simulink model "CAVE_MachE_dSPACE_250912"  (R2024a)
settings: configuration reference "ConfigSetDesktopFixedStep" (kept outside this file)
PreLoadFcn:
  | VSS_BICYCLE=Simulink.Variant('Dual=0');
  | VSS_DUAL=Simulink.Variant('Dual=1');
  | Dual=1;
  | load('DriveCycle2.mat')
PostLoadFcn:
  | if any(exist('dsrtsu_mdlpostloadfcn', 'file') ~= 0), dsrtsu_mdlpostloadfcn('Execute', bdroot); end
InitFcn:
  | , if any(exist('rtifpga_mdlclblib', 'file') ~= 0), rtifpga_mdlclblib('Init', bdroot); end,
  | , if any(exist('dsmpb_private', 'file') ~= 0), dsmpb_private('dsmpb_mdlclblib', 'Init', bdroot); end,
  | load('DriveCycle2.mat')
model workspace (MAT data in the model file):
  Gas = 0.383333333333
values from neighbouring files (symbols this model uses):
  CoastDown =     [Run_Simulink.mat]
  limitedMCT =     [Run_Simulink.mat]
  MCT =     [Run_Simulink.mat]
  pMCT =     [Run_Simulink.mat]
  RealSimPara =     [Run_Simulink.mat]
  Ref_speed = [13 13.007895099 13.015778396 13.023649891 13.031509584 13.039357475 13.047193564 13.055017851 13.062830336 13.070631019 13.0784199 13.086196979 ... (2669 elements, 2669x1)]    [Ref_speed_and_time.mat]
  Ref_time = [0 0.01 0.02 0.03 0.04 0.05 0.06 0.07 0.08 0.09 0.1 0.11 ... (2669 elements, 2669x1)]    [Ref_speed_and_time.mat]
  US06 =     [Run_Simulink.mat]
undefined symbols (not defined in the file or in its folder): AccelCmd, ActTqLF_Nm_, ActTqLR_Nm_, ActTqRF_Nm_, ActTqRR_Nm_, BattChargeLimitMaxPwr, BattChargeLimitSocBpts, BattChargeLimitTbl, BattChrgCapcty, BattDischargeLimitSocBpts, BattDischargeLimitTbl, BattDischargeMaxPwr, BattNumCellsParallel, BattNumCellsSeries, BattOpenVoltCapBpts, BattOpenVoltTbl, BattResistSocBpts, BattResistTbl, BattResistTempBpts, BrakeMaxPrs, BrakeMaxTrq, ChassisDistCg2FrontAxle, ChassisDistCg2RearAxle, ChassisVehMass, CltchCmd, DecelCmd, DiffRatio, DiscIntNeverNeededParam, EnvGravCnst, EnvPrs, EnvTemp, FuelSpecificGrav, GearCmd, h, InitStates, lgSw, MtrEffSpdBpts, MtrEffTbl, MtrEffTrqBpts, MtrPwrMax, MtrTrqMax, SteeringCmd, SupvsryCtrlRegenBrkCutOffTbl, SupvsryCtrlRegenSpdBpts, TestScnrioCycleNum, VEH
libraries: VSIGenLib x122, simulink x112, etargetslib x75, dsmpblib x55, vehdynlibtire x24, CarMaker4SL x20, autolibshared x19, vehdynlibsuspension x14, vehdynlibtirecommon x14, autolibutils x10, VsrLibWheel x8, autolibpowerinfoutils x6
(part 15 of 31)

== system CAVE_MachE_dSPACE_250912/Vehicle Under Test2/Vehicle/Vehicle Dynamics/Vehicle 7DOF/Longitudinal Wheels 4DOF/Tires ==
  AxlTrq : Inport
  BrkPrs : Inport  Port=2
  Vx : Inport  Port=3
  Vy : Inport  Port=4
  r : Inport  Port=5
  Camber : Inport  Port=6
  TirePrs : Inport  Port=7
  Fz : Inport  Port=8
  lam_mu : Inport  Port=9
  Gnd : Inport  Port=10
  4-by-1 Gnd : Subsystem
  4-by-1 Gnd1 : Subsystem
  4-by-1 Gnd2 : Subsystem
  4-by-1 Gnd3 : Subsystem
  Bus Creator : BusCreator  Inputs=12
  Subsystem : Subsystem
  Terminator1 : Terminator
  Terminator2 : Terminator
  Terminator3 : Terminator
  Wheel : Outport  VectorParamsAs1DForOutWhenUnconnected=off
  wires:
  Vy/1 -> Terminator1/1
  Camber/1 -> Terminator2/1
  r/1 -> Terminator3/1
  Bus Creator/1 -> Wheel/1
  Subsystem/7(zdot) -> Bus Creator/10  "zdot"
  Subsystem/6(z) -> Bus Creator/9  "z"
  Subsystem/2(Fx) -> Bus Creator/2  "Fx"
  Subsystem/1(Omega) -> Bus Creator/1  "Omega"
  Subsystem/5(Re) -> Bus Creator/8  "Re"
  Subsystem/3(FzOut) -> Bus Creator/4  "Fz"
  Subsystem/4(My) -> Bus Creator/6  "My"
  4-by-1 Gnd/1(Gnd) -> Bus Creator/3  "Fy"
  4-by-1 Gnd1/1(Gnd) -> Bus Creator/5  "Mx"
  4-by-1 Gnd2/1(Gnd) -> Bus Creator/7  "Mz"
  Subsystem/8(Kappa) -> Bus Creator/11  "Kappa"
  4-by-1 Gnd3/1(Gnd) -> Bus Creator/12  "Alpha"
  AxlTrq/1 -> Subsystem/1(AxlTrq)
  BrkPrs/1 -> Subsystem/2(BrkPrs)
  Vx/1 -> Subsystem/3(Vx)
  TirePrs/1 -> Subsystem/4(TirePrs)
  Fz/1 -> Subsystem/5(Fz)
  lam_mu/1 -> Subsystem/6(lam_mu)
  Gnd/1 -> Subsystem/7(Gnd)

== system CAVE_MachE_dSPACE_250912/Vehicle Under Test2/Vehicle/Vehicle Dynamics/Vehicle 7DOF/Longitudinal Wheels 4DOF/Veh2Tire ==
  AxlTrq : Inport
  BrkPrs : Inport  Port=2
  r : Inport  Port=3
  VehVel : Inport  Port=4
  WhlAng : Inport  Port=5
  Reshape3 : Reshape
  Reshape4 : Reshape
  Unary Minus : UnaryMinus
  Wheel to Body Transform : Subsystem
  T : Outport  VectorParamsAs1DForOutWhenUnconnected=off
  P : Outport  Port=2  VectorParamsAs1DForOutWhenUnconnected=off
  xdotAxle : Outport  Port=3  VectorParamsAs1DForOutWhenUnconnected=off
  ydotAxle : Outport  Port=4  VectorParamsAs1DForOutWhenUnconnected=off
  psidot : Outport  Port=5  VectorParamsAs1DForOutWhenUnconnected=off
  zdotAxle : Outport  Port=6  VectorParamsAs1DForOutWhenUnconnected=off
  wires:
  BrkPrs/1 -> Reshape3/1
  AxlTrq/1 -> Reshape4/1
  Wheel to Body Transform/1(xdotWheel) -> xdotAxle/1  "Vx"
  Wheel to Body Transform/2(ydotWheel) -> ydotAxle/1  "Vy"
  r/1 -> Unary Minus/1
  Reshape4/1 -> T/1
  VehVel/1 -> Wheel to Body Transform/1(VelVeh)
  WhlAng/1 -> Wheel to Body Transform/2(WhlAng)
  Wheel to Body Transform/3(zdotWheel) -> zdotAxle/1  "Vz"
  Unary Minus/1 -> psidot/1
  Reshape3/1 -> P/1

== system CAVE_MachE_dSPACE_250912/Vehicle Under Test2/Vehicle/Vehicle Dynamics/Vehicle 7DOF/Longitudinal Wheels 4DOF/Velocity and Vertical Load ==
  note: 1) Add Subsystem or Model blocks as valid variant choices.
      | 2) You cannot connect blocks at this level. At simulation, connectivity is automatically
      | determined, based on the active variant and port name matching.
  VehFdbk : Inport
  Bicycle : Subsystem  VariantControl=0
  Dual : Subsystem  VariantControl=1
  VehVel : Outport  VectorParamsAs1DForOutWhenUnconnected=off
  Fz : Outport  Port=2  PortDimensions=4  VectorParamsAs1DForOutWhenUnconnected=off

== system CAVE_MachE_dSPACE_250912/Vehicle Under Test2/Vehicle/Vehicle Dynamics/Vehicle 7DOF/Longitudinal Wheels 4DOF/Wheel Angles ==
  WheelAng : Inport
  Camber : Inport  Port=2
  Add1 : Sum
  Constant2 : Constant  Value=0
  Constant3 : Constant  Value=ones(1,4).*pi
  Demux : Demux  Outputs=2
  Demux1 : Demux
  Mux : Mux  Inputs=2
  Reshape : Reshape  OutputDimensionality=Row vector (2-D)
  Reshape1 : Reshape  OutputDimensionality=Row vector (2-D)
  Reshape2 : Reshape  OutputDimensionality=Row vector (2-D)
  Vector Concatenate3 : Concatenate  NumInputs=3  Mode=Multidimensional array
  Vector Concatenate4 : Concatenate  NumInputs=4
  WhlAngB : Outport  VectorParamsAs1DForOutWhenUnconnected=off
  wires:
  Demux1/2 -> Mux/1
  Constant2/1 -> Add1/2
  Add1/1 -> Demux/1
  Demux1/3 -> Vector Concatenate4/3
  Demux1/1 -> Vector Concatenate4/1
  Mux/1 -> Add1/1
  Demux1/4 -> Mux/2
  Demux/1 -> Vector Concatenate4/2
  Demux/2 -> Vector Concatenate4/4
  Vector Concatenate4/1 -> Reshape/1
  Constant3/1 -> Reshape1/1
  Vector Concatenate3/1 -> WhlAngB/1
  Reshape/1 -> Vector Concatenate3/3
  Reshape1/1 -> Vector Concatenate3/1
  Reshape2/1 -> Vector Concatenate3/2
  Camber/1 -> Reshape2/1
  WheelAng/1 -> Demux1/1

== system CAVE_MachE_dSPACE_250912/Vehicle Under Test2/Vehicle/Vehicle Dynamics/Vehicle 7DOF/Subsystem4/Subsystem ==
  CgXYZdot : Inport
  angles : Inport  Port=2
  Demux2 : Demux  Outputs=3
  Demux3 : Demux  Outputs=3
  Terminator{,1..4} (5 alike) : Terminator
  VehSpd : Outport
  wires:
  CgXYZdot/1 -> Demux2/1
  Demux3/2 -> Terminator3/1  "theta"
  Demux2/2 -> Terminator/1  "Ydot"
  Demux3/1 -> Terminator2/1  "phi"
  Demux3/3 -> Terminator4/1  "psi"
  Demux2/3 -> Terminator1/1  "Zdot"
  angles/1 -> Demux3/1
  Demux2/1 -> VehSpd/1  "Xdot"

== system CAVE_MachE_dSPACE_250912/Vehicle Under Test2/Vehicle/Vehicle Dynamics/Vehicle 7DOF/Vehicle Body 3DOF External Longitudinal Wheels/Bicycle ==
  WhlAng : Inport
  "FwF " : Inport  Port=2
  "FwR " : Inport  Port=3
  WindXYZ : Inport  Port=4
  Friction : Inport  Port=5
  Demux : Demux  Outputs=[2,2]
  Gain : Gain  Gain=.5
  Gain1 : Gain  Gain=.5
  Gain2 : Gain  Gain=.5
  Selector : Selector  InputPortWidth=4  IndexOptions=Index vector (dialog)  Indices=[1 2]  OutputSizes=1
  Signal Specification : SignalSpecification  Unit=1
  Signal Specification1 : SignalSpecification  Unit=rad
  Sum of Elements : Sum  Inputs=+
  Sum of Elements1 : Sum  Inputs=+
  Sum of Elements2 : Sum  Inputs=+
  Terminator{,1..5} (6 alike) : Terminator
  Vector Concatenate : Concatenate
  Vehicle Body 3DOF Single Track : autolibshared/Vehicle Body 3DOF Single Track  trackMode=Single (bicycle)  inputMode=External longitudinal forces  frontSteerMode=on  rearSteerMode=off  windMode=on  muMode=on  extFMode=off  extMMode=off  htchFMode=off  htchMMode=off  extXo=off  extpsio=off  extxdoto=off  extro=off  extYo=off  extTamb=off  extydoto=off  aMode=2  NF=ChassisNumFrontWhls  NR=ChassisNumRearWhls  m=ChassisVehMass  a=ChassisDistCg2FrontAxle  b=ChassisDistCg2RearAxle  h=ChassisCgHeight  dh=1  hh=0.2  X_o=0  xdot_o=20  CalphaMode=off  sigmaMode=on  d=0  hl=0  w=1.922.*[1 1]  Cy_f=15000  Cy_r=35000  sigma_f=.1  sigma_r=.1  alpha_f_brk=[-.1 .1]  Cy_f_data=[-9e3 9e3]  alpha_r_brk=[-.1 .1]  Cy_r_data=[-9e3 9e3]  Y_o=0  ydot_o=0  Izz=2500  psi_o=0  r_o=0  Af=ChassisFrontalArea  Cd=ChassisDragCoeff  Cl=.1  Cpm=.1  beta_w=[0:0.01:0.3]  Cs=[0:0.03:0.9]  Cym=[0:0.01:0.3]  Pabs=EnvPrs  Tair=EnvTemp  g=EnvGravCnst  mu=1  xdot_tol=1  Fznom=5000  Fxtire_sat=7e3*1e3  Fytire_sat=2e3*1e3  longOff=0  latOff=0  vertOff=.0112  wrapAng=off
  Wheel Positions : Subsystem
  " Info" : Outport  VectorParamsAs1DForOutWhenUnconnected=off
  XWheel : Outport  Port=2  Unit=m  VectorParamsAs1DForOutWhenUnconnected=off
  " YWheel" : Outport  Port=3  Unit=m  VectorParamsAs1DForOutWhenUnconnected=off
  wires:
  "FwR "/1 -> Vehicle Body 3DOF Single Track/3
  "FwF "/1 -> Vehicle Body 3DOF Single Track/2
  Vehicle Body 3DOF Single Track/1 -> " Info"/1, Wheel Positions/1(Info)
  WhlAng/1 -> Selector/1
  Gain/1 -> Signal Specification1/1
  Sum of Elements/1 -> Gain/1
  Vehicle Body 3DOF Single Track/6 -> Terminator/1
  Vehicle Body 3DOF Single Track/7 -> Terminator1/1
  WindXYZ/1 -> ?
  Selector/1 -> Sum of Elements/1
  Demux/1 -> Sum of Elements1/1
  Friction/1 -> Demux/1
  Sum of Elements1/1 -> Gain1/1
  Sum of Elements2/1 -> Gain2/1
  Demux/2 -> Sum of Elements2/1
  Gain1/1 -> Vector Concatenate/1
  Gain2/1 -> Vector Concatenate/2
  Vector Concatenate/1 -> Signal Specification/1
  Signal Specification/1 -> ?
  Signal Specification1/1 -> Vehicle Body 3DOF Single Track/1
  Wheel Positions/2(YWheel) -> " YWheel"/1
  Wheel Positions/1(XWheel) -> XWheel/1
  Vehicle Body 3DOF Single Track/4 -> Terminator2/1
  Vehicle Body 3DOF Single Track/5 -> Terminator3/1
  Vehicle Body 3DOF Single Track/2 -> Terminator4/1
  Vehicle Body 3DOF Single Track/3 -> Terminator5/1

== system CAVE_MachE_dSPACE_250912/Vehicle Under Test2/Vehicle/Vehicle Dynamics/Vehicle 7DOF/Vehicle Body 3DOF External Longitudinal Wheels/Dual ==
  WhlAng : Inport
  "FwF " : Inport  Port=2
  "FwR " : Inport  Port=3
  WindXYZ : Inport  Port=4
  Friction : Inport  Port=5
  Reshape : Reshape  OutputDimensionality=Customize  OutputDimensions=[2,2]
  Selector : Selector  InputPortWidth=4  IndexOptions=Index vector (dialog)  Indices=[1 2]  OutputSizes=1
  Signal Specification : SignalSpecification  Unit=1
  Terminator{,1..5} (6 alike) : Terminator
  Vehicle Body 3DOF Dual Track : autolibshared/Vehicle Body 3DOF Single Track  trackMode=Dual  inputMode=External longitudinal forces  frontSteerMode=on  rearSteerMode=off  windMode=on  muMode=on  extFMode=off  extMMode=off  htchFMode=off  htchMMode=off  extXo=off  extpsio=off  extxdoto=off  extro=off  extYo=off  extTamb=off  extydoto=off  aMode=2  NF=ChassisNumFrontWhls  NR=ChassisNumRearWhls  m=ChassisVehMass  a=ChassisDistCg2FrontAxle  b=ChassisDistCg2RearAxle  h=ChassisCgHeight  dh=1  hh=0.2  X_o=0  xdot_o=InitStates(TestScnrioCycleNum).VehSpd  CalphaMode=off  sigmaMode=on  d=0  hl=0  w=1.9.*[1 1]  Cy_f=15000  Cy_r=35000  sigma_f=.1  sigma_r=.1  alpha_f_brk=[-.1 .1]  Cy_f_data=[-9e3 9e3]  alpha_r_brk=[-.1 .1]  Cy_r_data=[-9e3 9e3]  Y_o=0  ydot_o=0  Izz=2500  psi_o=0  r_o=0  Af=ChassisFrontalArea  Cd=ChassisDragCoeff  Cl=.1  Cpm=.1  beta_w=[0:0.01:0.3]  Cs=[0:0.03:0.9]  Cym=[0:0.01:0.3]  Pabs=EnvPrs  Tair=EnvTemp  g=EnvGravCnst  mu=1  xdot_tol=1  Fznom=5000  Fxtire_sat=7e3*1e3  Fytire_sat=2e3*1e3  longOff=0  latOff=0  vertOff=.0112  wrapAng=off
  Wheel Positions : Subsystem
  " Info" : Outport  VectorParamsAs1DForOutWhenUnconnected=off
  " XWheel" : Outport  Port=2  VectorParamsAs1DForOutWhenUnconnected=off
  " YWheel" : Outport  Port=3  VectorParamsAs1DForOutWhenUnconnected=off
  wires:
  WhlAng/1 -> Selector/1
  Selector/1 -> Vehicle Body 3DOF Dual Track/1
  Friction/1 -> Reshape/1
  Reshape/1 -> Signal Specification/1
  Vehicle Body 3DOF Dual Track/1 -> " Info"/1, Wheel Positions/1(Info)
  Wheel Positions/1(XWheel) -> " XWheel"/1
  Wheel Positions/2(YWheel) -> " YWheel"/1
  Vehicle Body 3DOF Dual Track/2 -> Terminator4/1
  Vehicle Body 3DOF Dual Track/3 -> Terminator5/1
  Vehicle Body 3DOF Dual Track/6 -> Terminator1/1
  Vehicle Body 3DOF Dual Track/4 -> Terminator2/1
  Vehicle Body 3DOF Dual Track/5 -> Terminator3/1
  Vehicle Body 3DOF Dual Track/7 -> Terminator/1
  Signal Specification/1 -> ?
  WindXYZ/1 -> ?
  "FwF "/1 -> Vehicle Body 3DOF Dual Track/2
  "FwR "/1 -> Vehicle Body 3DOF Dual Track/3

== system CAVE_MachE_dSPACE_250912/Vehicle Under Test2/Vehicle/Vehicle Dynamics/Vehicle Longitudinal/Longitudinal Wheels/Front Diff Wheels ==
  BrkPrs : Inport
  AxleTorq : Inport  Port=2
  Add2 : Sum
  Bus Creator : BusCreator  Inputs=3
  Bus Creator5 : BusCreator  Inputs=1
  Bus Selector6 : BusSelector  OutputSignals=VehSpd,FrcZ
  Bus Selector7 : BusSelector  OutputSignals=VehSpd,FrcZ
  Selector : Selector  InputPortWidth=4  IndexOptions=Index vector (dialog)  Indices=1  OutputSizes=1
  Selector1 : Selector  InputPortWidth=4  IndexOptions=Index vector (dialog)  Indices=2  OutputSizes=1
  Selector2 : Selector  InputPortWidth=4  IndexOptions=Index vector (dialog)  Indices=1  OutputSizes=1
  Selector3 : Selector  InputPortWidth=4  IndexOptions=Index vector (dialog)  Indices=2  OutputSizes=1
  Simple Longitudinal Wheel 1 : VsrLibWheel/Simple Longitudinal Wheel  TireLoadedRadius=WhlRearLoadedRadius  C_rr=WhlRollingResistCnst  MaxBrkTrq=BrakeMaxTrq  MaxBrkPrs=BrakeMaxPrs  w_thresh=WhlSimVelTol
  Simple Longitudinal Wheel 2 : VsrLibWheel/Simple Longitudinal Wheel  TireLoadedRadius=WhlRearLoadedRadius  C_rr=WhlRollingResistCnst  MaxBrkTrq=BrakeMaxTrq  MaxBrkPrs=BrakeMaxPrs  w_thresh=WhlSimVelTol
  Terminator3 : Terminator
  Two-Way Connection6 : TwoWayConnection
  DiffAxle : PMIOPort  Side=Right
  Info : Outport
  wires:
  Bus Selector6/2 -> Simple Longitudinal Wheel 1/4  "<FrcZ>"
  BrkPrs/1 -> Selector3/1, Selector2/1
  Simple Longitudinal Wheel 1/2 -> Add2/1
  Bus Selector7/1 -> Simple Longitudinal Wheel 2/3  "<VehSpd>"
  Bus Selector6/1 -> Simple Longitudinal Wheel 1/3  "<VehSpd>"
  Bus Selector7/2 -> Simple Longitudinal Wheel 2/4  "<FrcZ>"
  Two-Way Connection6/1 -> Bus Selector7/1, Bus Selector6/1
  Add2/1 -> Bus Creator5/1  "FrcX"
  Simple Longitudinal Wheel 2/2 -> Add2/2  "Spd"
  Bus Creator5/1 -> Two-Way Connection6/1
  Simple Longitudinal Wheel 2/1 -> Terminator3/1
  Selector2/1 -> Simple Longitudinal Wheel 1/1
  AxleTorq/1 -> Selector1/1, Selector/1
  Selector/1 -> Simple Longitudinal Wheel 1/2
  Selector1/1 -> Simple Longitudinal Wheel 2/2
  Selector3/1 -> Simple Longitudinal Wheel 2/1
  Simple Longitudinal Wheel 1/3 -> Bus Creator/2  "Omega1"
  Bus Creator/1 -> Info/1
  Simple Longitudinal Wheel 1/1 -> Bus Creator/1  "WhlFrontInfo"
  Simple Longitudinal Wheel 2/3 -> Bus Creator/3  "Omega2"
  connections:
  DiffAxle/RConn1 -- Two-Way Connection6/RConn1

== system CAVE_MachE_dSPACE_250912/Vehicle Under Test2/Vehicle/Vehicle Dynamics/Vehicle Longitudinal/Longitudinal Wheels/Rear Wheels ==
  BrkPrs : Inport
  Add2 : Sum
  Bus Creator : BusCreator  Inputs=3
  Bus Creator5 : BusCreator  Inputs=1
  Bus Selector6 : BusSelector  OutputSignals=VehSpd,FrcZ
  Bus Selector7 : BusSelector  OutputSignals=VehSpd,FrcZ
  Ground : Ground
  Selector : Selector  InputPortWidth=4  IndexOptions=Index vector (dialog)  Indices=3  OutputSizes=1
  Selector1 : Selector  InputPortWidth=4  IndexOptions=Index vector (dialog)  Indices=4  OutputSizes=1
  Simple Longitudinal Wheel : VsrLibWheel/Simple Longitudinal Wheel  TireLoadedRadius=WhlFrontLoadedRadius  C_rr=WhlRollingResistCnst  MaxBrkTrq=BrakeMaxTrq  MaxBrkPrs=BrakeMaxPrs  w_thresh=WhlSimVelTol
  Simple Longitudinal Wheel1 : VsrLibWheel/Simple Longitudinal Wheel  TireLoadedRadius=WhlFrontLoadedRadius  C_rr=WhlRollingResistCnst  MaxBrkTrq=BrakeMaxTrq  MaxBrkPrs=BrakeMaxPrs  w_thresh=WhlSimVelTol
  Terminator3 : Terminator
  Two-Way Connection6 : TwoWayConnection
  DiffAxle : PMIOPort  Side=Right
  Info : Outport
  wires:
  Simple Longitudinal Wheel1/1 -> Terminator3/1
  Simple Longitudinal Wheel1/3 -> Bus Creator/3  "Omega4"
  Ground/1 -> Simple Longitudinal Wheel/2, Simple Longitudinal Wheel1/2
  Simple Longitudinal Wheel/3 -> Bus Creator/2  "Omega3"
  Bus Creator5/1 -> Two-Way Connection6/1
  Simple Longitudinal Wheel1/2 -> Add2/2  "Spd"
  Add2/1 -> Bus Creator5/1  "FrcX"
  Two-Way Connection6/1 -> Bus Selector7/1, Bus Selector6/1
  Bus Selector7/2 -> Simple Longitudinal Wheel1/4  "<FrcZ>"
  Bus Selector6/1 -> Simple Longitudinal Wheel/3  "<VehSpd>"
  Bus Selector7/1 -> Simple Longitudinal Wheel1/3  "<VehSpd>"
  Simple Longitudinal Wheel/2 -> Add2/1
  BrkPrs/1 -> Selector1/1, Selector/1
  Bus Selector6/2 -> Simple Longitudinal Wheel/4  "<FrcZ>"
  Selector/1 -> Simple Longitudinal Wheel/1
  Selector1/1 -> Simple Longitudinal Wheel1/1
  Simple Longitudinal Wheel/1 -> Bus Creator/1  "WhlRearInfo"
  Bus Creator/1 -> Info/1
  connections:
  DiffAxle/RConn1 -- Two-Way Connection6/RConn1

== system CAVE_MachE_dSPACE_250912/Vehicle Under Test2/Vehicle/Vehicle Dynamics/Vehicle Longitudinal/Vehicle Body/Logitudinal Vehicle Body ==
  RoadGrade : Inport
  WindVel : Inport  Port=2  Unit=m/s
  Bus Creator : BusCreator  Inputs=2
  Bus Creator1 : BusCreator  Inputs=2
  Bus Selector : BusSelector  OutputSignals=FrcX
  Bus Selector1 : BusSelector  OutputSignals=BdyFrm.Cg.Vel.xdot,BdyFrm.Cg.Disp.x
  Bus Selector3 : BusSelector  OutputSignals=FrcX
  Signal Specification3 : SignalSpecification  Unit=N
  Signal Specification4 : SignalSpecification  Unit=N
  Transfer Fcn : TransferFcn  Denominator=[0.01 1]
  Transfer Fcn1 : TransferFcn  Denominator=[0.01 1]
  Two-Way Connection2 : TwoWayConnection
  Two-Way Connection8 : TwoWayConnection
  Unit Conversion : UnitConversion
  Vehicle Body 1DOF Longitudinal : autolibshared/Vehicle Body 1DOF Longitudinal  VariantControl=SL  extFMode=off  extMMode=off  extTamb=off  wind3D=off  aMode=1  NF=ChassisNumFrontWhls  NR=ChassisNumRearWhls  m=ChassisVehMass  a=ChassisDistCg2FrontAxle  b=ChassisDistCg2RearAxle  h=ChassisCgHeight  Cd=ChassisDragCoeff  Cl=0  Cpm=0  Af=ChassisFrontalArea  x_o=0  xdot_o=InitStates(TestScnrioCycleNum).VehSpd  Pabs=EnvPrs  T=EnvTemp  g=EnvGravCnst
      settings: LibrarySourceBlock=autolibvehdynlong/Vehicle Body 1DOF Longitudinal
  Front : PMIOPort  Side=Left
  Rear : PMIOPort  Port=2  Side=Left
  VehSpd : Outport  VectorParamsAs1DForOutWhenUnconnected=off
  VehDist : Outport  Port=2  VectorParamsAs1DForOutWhenUnconnected=off
  FrontAxleFrc : Outport  Port=3  VectorParamsAs1DForOutWhenUnconnected=off
  RearAxleFrc : Outport  Port=4  VectorParamsAs1DForOutWhenUnconnected=off
  wires:
  Two-Way Connection8/1 -> Bus Selector/1
  RoadGrade/1 -> Unit Conversion/1
  Bus Selector/1 -> Transfer Fcn1/1  "<FrcX>"
  Vehicle Body 1DOF Longitudinal/2 -> Bus Creator/1, Bus Creator1/1  "VehSpd"
  Vehicle Body 1DOF Longitudinal/1 -> Bus Selector1/1  "Veh"
  Signal Specification3/1 -> RearAxleFrc/1, Vehicle Body 1DOF Longitudinal/2  "RearAxleFrc"
  Bus Creator/1 -> Two-Way Connection8/1
  Vehicle Body 1DOF Longitudinal/3 -> Bus Creator/2  "FrcZ"
  WindVel/1 -> Vehicle Body 1DOF Longitudinal/4
  Two-Way Connection2/1 -> Bus Selector3/1
  Vehicle Body 1DOF Longitudinal/4 -> Bus Creator1/2  "FrcZ"
  Bus Selector1/1 -> VehSpd/1  "<xdot>"
  Bus Selector1/2 -> VehDist/1  "<x>"
  Unit Conversion/1 -> Vehicle Body 1DOF Longitudinal/3
  Signal Specification4/1 -> FrontAxleFrc/1, Vehicle Body 1DOF Longitudinal/1  "FrontAxleFrc"
  Transfer Fcn/1 -> Signal Specification3/1
  Transfer Fcn1/1 -> Signal Specification4/1
  Bus Creator1/1 -> Two-Way Connection2/1
  Bus Selector3/1 -> Transfer Fcn/1  "<FrcX>"
  connections:
  Two-Way Connection8/RConn1 -- Front/RConn1
  Two-Way Connection2/RConn1 -- Rear/RConn1

== system CAVE_MachE_dSPACE_250912/Vehicle Under Test2/Vehicle/Vehicle Dynamics/Vehicle Longitudinal/Vehicle Body/Subsystem1 ==
  VehSpd : Inport
  VehDist : Inport  Port=2
  FrontAxleFrc : Inport  Port=3
  RearAxleFrc : Inport  Port=4
  Bus Creator : BusCreator  Inputs=4
  ChassisPlant : Outport
  wires:
  VehSpd/1 -> Bus Creator/1  "VehSpd"
  VehDist/1 -> Bus Creator/2  "VehDist"
  Bus Creator/1 -> ChassisPlant/1  "ChassisPlant"
  FrontAxleFrc/1 -> Bus Creator/3  "FrontAxleFrc"
  RearAxleFrc/1 -> Bus Creator/4  "RearAxleFrc"

== system CAVE_MachE_dSPACE_250912/Vehicle Under Test3/Vehicle/Actuation and Outputs/MOOG Brake Actuator/ CAN Settings/ CAN diagnostic Counter ==
  RX Counter : Inport
  Compare To Constant3 : simulink/Logic and Bit Operations/Compare To Constant  relop=<=  const=TimeOutDuration  OutDataTypeStr=boolean
  Memory2 : Memory  InheritSampleTime=on
  Relational Operator2 : RelationalOperator  Operator=~=  OutDataTypeStr=boolean  InputSameDT=off
  Timer : Subsystem
  CommsOKFlag : Outport
  wires:
  Relational Operator2/1 -> Timer/1(Reset)
  Timer/1(Timer) -> Compare To Constant3/1
  RX Counter/1 -> Relational Operator2/1, Memory2/1
  Memory2/1 -> Relational Operator2/2
  Compare To Constant3/1 -> CommsOKFlag/1

== system CAVE_MachE_dSPACE_250912/Vehicle Under Test3/Vehicle/Actuation and Outputs/MOOG Brake Actuator/MOOG Interface/Max Stop Adjustment ==
  In1 : Inport
  Enable : EnablePort
  MaxStopOffset : Constant  Value=-5500
  Sum3 : Sum  Inputs=|++
  Out1 : Outport  InitialOutput=[0]
  wires:
  MaxStopOffset/1 -> Sum3/2
  In1/1 -> Sum3/1
  Sum3/1 -> Out1/1

== system CAVE_MachE_dSPACE_250912/Vehicle Under Test3/Vehicle/Actuation and Outputs/MOOG Brake Actuator/MOOG Interface/Min Stop Adjustment ==
  In1 : Inport
  Enable : EnablePort
  MinStopOffset : Constant  Value=3500
  Sum3 : Sum  Inputs=|++
  Out1 : Outport  InitialOutput=[0]
  wires:
  In1/1 -> Sum3/1
  Sum3/1 -> Out1/1
  MinStopOffset/1 -> Sum3/2

== system CAVE_MachE_dSPACE_250912/Vehicle Under Test3/Vehicle/Actuation and Outputs/MOOG Brake Actuator/MOOG Interface/Rising edge ==
  In : Inport
  Memory : Memory  InheritSampleTime=on
  Sum3 : Sum  Inputs=|+-
  Out : Outport
  wires:
  In/1 -> Memory/1, Sum3/1
  Memory/1 -> Sum3/2
  Sum3/1 -> Out/1

== system CAVE_MachE_dSPACE_250912/Vehicle Under Test3/Vehicle/Actuation and Outputs/MOOG Brake Actuator/MOOG Interface/Rising edge1 ==
  In : Inport
  Memory : Memory  InheritSampleTime=on
  Sum3 : Sum  Inputs=|+-
  Out : Outport
  wires:
  In/1 -> Memory/1, Sum3/1
  Memory/1 -> Sum3/2
  Sum3/1 -> Out/1

== system CAVE_MachE_dSPACE_250912/Vehicle Under Test3/Vehicle/Battery/Battery/Lithium Ion Battery Pack1/Datasheet Battery Internal ==
  BattCurr : Inport
  BattTemp : Inport  Port=2
  Constant1 : Constant  Value=BattCapInit
  Datasheet Battery : Subsystem  AncestorBlock=autolibbatterycommon/Datasheet Battery
  LdCurrFeed : Outport  VectorParamsAs1DForOutWhenUnconnected=off
  OutVoltUnfilt : Outport  Port=2  VectorParamsAs1DForOutWhenUnconnected=off
  LdAmpHr : Outport  Port=3  VectorParamsAs1DForOutWhenUnconnected=off
  BattSoc : Outport  Port=4  VectorParamsAs1DForOutWhenUnconnected=off
  BattPwrLoss : Outport  Port=5  VectorParamsAs1DForOutWhenUnconnected=off
  wires:
  Datasheet Battery/5(BattPwrLoss) -> BattPwrLoss/1
  Datasheet Battery/1(LdCurrFeed) -> LdCurrFeed/1
  Datasheet Battery/2(OutVoltUnfilt) -> OutVoltUnfilt/1
  Datasheet Battery/3(LdAmpHr) -> LdAmpHr/1
  Datasheet Battery/4(BattSoc) -> BattSoc/1
  BattTemp/1 -> Datasheet Battery/3(BattTemp)
  BattCurr/1 -> Datasheet Battery/2(BattCurr)
  Constant1/1 -> Datasheet Battery/1(CapInit)

== system CAVE_MachE_dSPACE_250912/Vehicle Under Test3/Vehicle/Driver and Drive Cycle/Driver and PI with FF Control/Speed controller set/In-house CAVE ==
  note: BrakeSwitch
  RefSpd [km/hr] : Inport
  In2 : Inport  Port=2
  In-house Speed Controller : Subsystem
  AccelPedalCmd : Outport
  BrakePedalCmd : Outport  Port=2
  Out3 : Outport  Port=3
  wires:
  In-house Speed Controller/3(BrakeSwitch) -> Out3/1
  In-house Speed Controller/2(BrakePedalPos) -> BrakePedalCmd/1  "BrakePedalCmd"
  RefSpd [km/hr]/1 -> In-house Speed Controller/1(RefSpd)
  In2/1 -> In-house Speed Controller/2(VehicleSpeed)
  In-house Speed Controller/1(AcceleratorPedalPos) -> AccelPedalCmd/1  "AccelPedalCmd"

== system CAVE_MachE_dSPACE_250912/Vehicle Under Test3/Vehicle/Driver and Drive Cycle/Driver and PI with FF Control/Speed controller set/PIF ==
  RefSpd [km/hr] : Inport
  In2 : Inport  Port=2
  Compare To Constant1 : simulink/Logic and Bit Operations/Compare To Constant  relop=<=  const=0.1  OutDataTypeStr=boolean  ZeroCross=off
  Constant : Constant  Value=0
  Constant1 : Constant  Value=0
  Gain : Gain  Gain=1/3.6
  Gain1 : Gain  Gain=1/3.6
  Gain2 : Gain  Gain=100
  Gain3 : Gain  Gain=100
  Longitudinal Driver : autolibshared/Longitudinal Driver  extAccelOvr=off  extDecelOvr=off  extAccelHld=off  extDecelHld=off  extAccelZero=off  extDecelZero=off  cntrlType=PI  shftType=None  velUnits=m/s  gearOut=off  Kp=2.5  Ki=1  Kff=.1*0.35  Kg=0  VehVelVec=[0 100]  KffVec=[.1 .1]  KpVec=[10 10]  KiVec=[5 5]  KgVec=[0 0]  m=1500  Kpt=3000  tau=.1  L=2  aR=200  bR=2.5  cR=.5  g=9.81  vnom=1  Kaw=1  tauerr=.01  tauPt=2  GearInit=0  tShift=.1  pdlVec=[0.1 0.4 0.5 0.9]  upShftTbl=[-1 12.9375 26.4375 39.9375 51.18749999999999 62.4375 72.84375 83.25;-1 16.3125 29.8125 43.3125 54.5624 65.8125 76.78125 87.75;-1 19.6875 33.1875 46.68749999999999 57.9375 69.1875 80.71875 92.25;-1 33 52.5 77.25 100.5 138.75 161.875 185]  dwnShftTbl=[1 9.5625 23.0625 36.5625 47.8125 59.0625 68.90625 78.75;1 12.9375 26.4375 39.9375 51.18749999999999 62.4375 72.84375 83.25;1 16.3125 29.8125 43.3125 54.562499 65.8125 76.78125 87.75;1 19.6875 33.1875 46.68749999999999 57.9375 69.1875 80.71875 92.25]  tClutch=.5  tRev=.5  tPark=120  aMode=2  UpGearVec="[0  1  2  3  4  5  6  7]"  DownGearVec="[1  2  3  4  5  6  7  8]"
      settings: LibrarySourceBlock=vehdynlibdriver/Longitudinal Driver
  Lowpass Filter : TransferFcn  Denominator=[.01 1]
  Min threshold for Brake switch : Constant  Value=0
  Relational Operator : RelationalOperator  Operator=>  OutDataTypeStr=boolean  InputSameDT=off
  Switch3 : Switch  Criteria=u2 > Threshold  SaturateOnIntegerOverflow=off  InputSameDT=off
  Switch4 : Switch  Criteria=u2 > Threshold  SaturateOnIntegerOverflow=off  InputSameDT=off
  Terminator : Terminator
  standstill brake [0,1] : Constant  Value=0.5
  AccelPedalCmd : Outport
  BrakePedalCmd : Outport  Port=2
  Out3 : Outport  Port=3
  wires:
  Gain1/1 -> Longitudinal Driver/2
  Min threshold for Brake switch/1 -> Relational Operator/2
  Relational Operator/1 -> Out3/1  "BrakeSwitch"
  Longitudinal Driver/3 -> Switch4/3, Relational Operator/1  "BrakePedalPosPre_pct"
  Gain/1 -> Compare To Constant1/1, Longitudinal Driver/1
  Constant1/1 -> Longitudinal Driver/3
  RefSpd [km/hr]/1 -> Gain/1
  In2/1 -> Lowpass Filter/1
  Gain3/1 -> BrakePedalCmd/1  "BrakePedalCmd"
  Gain2/1 -> AccelPedalCmd/1  "AccelPedalCmd"
  Longitudinal Driver/1 -> Terminator/1
  Longitudinal Driver/2 -> Switch3/3  "AcceleratorPedalPosPre_pct"
  Constant/1 -> Switch3/1
  Compare To Constant1/1 -> Switch4/2, Switch3/2
  standstill brake [0,1]/1 -> Switch4/1
  Switch3/1 -> Gain2/1  "AcceleratorPedalPos_pct"
  Switch4/1 -> Gain3/1  "BrakePedalPos_pct"
  Lowpass Filter/1 -> Gain1/1  "VS_Flt"

== system CAVE_MachE_dSPACE_250912/Vehicle Under Test3/Vehicle/Driver and Drive Cycle/Driver and PI with FF Control/Speed controller set/Predictive ==
  RefSpd [km/hr] : Inport
  In2 : Inport  Port=2
  Compare To Constant1 : simulink/Logic and Bit Operations/Compare To Constant  relop=<=  const=0.1  OutDataTypeStr=boolean  ZeroCross=off
  Constant : Constant  Value=0
  Constant1 : Constant  Value=0
  Gain : Gain  Gain=1/3.6
  Gain1 : Gain  Gain=1/3.6
  Gain4 : Gain  Gain=100
  Gain5 : Gain  Gain=100
  Longitudinal Driver : autolibshared/Longitudinal Driver  extAccelOvr=off  extDecelOvr=off  extAccelHld=off  extDecelHld=off  extAccelZero=off  extDecelZero=off  cntrlType=Predictive  shftType=None  velUnits=m/s  gearOut=off  Kp=10  Ki=5  Kff=.1  Kg=0  VehVelVec=[0 100]  KffVec=[.1 .1]  KpVec=[10 10]  KiVec=[5 5]  KgVec=[0 0]  m=2040  Kpt=6500  tau=0.1  L=3  aR=200/10  bR=2.5/100  cR=.3  g=9.807  vnom=5  Kaw=1  tauerr=.01  tauPt=2  GearInit=0  tShift=.1  pdlVec=[0.1 0.4 0.5 0.9]  upShftTbl=[-1 12.9375 26.4375 39.9375 51.18749999999999 62.4375 72.84375 83.25;-1 16.3125 29.8125 43.3125 54.5624 65.8125 76.78125 87.75;-1 19.6875 33.1875 46.68749999999999 57.9375 69.1875 80.71875 92.25;-1 33 52.5 77.25 100.5 138.75 161.875 185]  dwnShftTbl=[1 9.5625 23.0625 36.5625 47.8125 59.0625 68.90625 78.75;1 12.9375 26.4375 39.9375 51.18749999999999 62.4375 72.84375 83.25;1 16.3125 29.8125 43.3125 54.562499 65.8125 76.78125 87.75;1 19.6875 33.1875 46.68749999999999 57.9375 69.1875 80.71875 92.25]  tClutch=.5  tRev=.5  tPark=120  aMode=2  UpGearVec="[0  1  2  3  4  5  6  7]"  DownGearVec="[1  2  3  4  5  6  7  8]"
      settings: LibrarySourceBlock=vehdynlibdriver/Longitudinal Driver
  Lowpass Filter : TransferFcn  Denominator=[.02 1]
  Min threshold for Brake switch : Constant  Value=0
  Relational Operator : RelationalOperator  Operator=>  OutDataTypeStr=boolean  InputSameDT=off
  Switch3 : Switch  Criteria=u2 > Threshold  SaturateOnIntegerOverflow=off  InputSameDT=off
  Switch4 : Switch  Criteria=u2 > Threshold  SaturateOnIntegerOverflow=off  InputSameDT=off
  Terminator : Terminator
  standstill brake [0,1] : Constant  Value=0.5
  AccelPedalCmd : Outport
  BrakePedalCmd : Outport  Port=2
  Out3 : Outport  Port=3
  wires:
  Gain1/1 -> Longitudinal Driver/2
  Min threshold for Brake switch/1 -> Relational Operator/2
  Relational Operator/1 -> Out3/1  "BrakeSwitch"
  Constant1/1 -> Longitudinal Driver/3
  RefSpd [km/hr]/1 -> Gain/1
  In2/1 -> Lowpass Filter/1
  Longitudinal Driver/1 -> Terminator/1
  standstill brake [0,1]/1 -> Switch4/1
  Longitudinal Driver/3 -> Switch4/3, Relational Operator/1  "BrakePedalPosPre_pct"
  Switch4/1 -> Gain5/1  "BrakePedalPos_pct"
  Switch3/1 -> Gain4/1  "AcceleratorPedalPos_pct"
  Compare To Constant1/1 -> Switch4/2, Switch3/2
  Constant/1 -> Switch3/1
  Gain4/1 -> AccelPedalCmd/1  "AccelPedalCmd"
  Gain/1 -> Compare To Constant1/1, Longitudinal Driver/1
  Gain5/1 -> BrakePedalCmd/1  "BrakePedalCmd"
  Longitudinal Driver/2 -> Switch3/3  "AcceleratorPedalPosPre_pct"
  Lowpass Filter/1 -> Gain1/1  "VS_Flt"

== system CAVE_MachE_dSPACE_250912/Vehicle Under Test3/Vehicle/Driver and Drive Cycle/Driver and PI with FF Control/Speed controller set/Speed tracking controller ==
  RefSpd [km/hr] : Inport
  In2 : Inport  Port=2
  In-house CAVE : Subsystem  VariantControl=varaint1
  PIF : Subsystem  VariantControl=varaint2
  Predictive : Subsystem  VariantControl=varaint3
  AccelPedalCmd : Outport
  BrakePedalCmd : Outport  Port=2
  Out3 : Outport  Port=3

== system CAVE_MachE_dSPACE_250912/Vehicle Under Test3/Vehicle/Powertrain Supervisory Controller /Engine Torque Command/Accel Pedal to Traction Wheel Torque Request1/Max Motor Torque ==
  MtrSpd : Inport
  Constant : Constant  Value=MtrPwrMax
  Divide : Product  Inputs=*/
  Saturation : Saturate  UpperLimit=MtrTrqMax  LowerLimit=0
  Saturation1 : Saturate  UpperLimit=inf  LowerLimit=1
  MtrTrqMax : Outport
  wires:
  Saturation/1 -> MtrTrqMax/1
  Saturation1/1 -> Divide/2
  Divide/1 -> Saturation/1
  MtrSpd/1 -> Saturation1/1
  Constant/1 -> Divide/1

== system CAVE_MachE_dSPACE_250912/Vehicle Under Test3/Vehicle/Powertrain Supervisory Controller /Engine Torque Command/Motor Torque Arbitration and Power Management/Power Management ==
  note: Power Management algorithm:
      | - Estimate Elec power based on mech power using efficiency map
      | - Check if Elec power is within battery power limits
      | - If power within limit , use motor torque command
      | - If power limit exceeded, use limited motor torque
      | - For low Mot Spd, MotPwrReq will be a small number.  Pass through torque command until Mot Spd > 2.
  BattPwrDischrgLmt : Inport
  BattPwrChrgLmt : Inport  Port=2
  MotSpd : Inport  Port=3
  MotTrqCmd : Inport  Port=4
  Abs : Abs  SaturateOnIntegerOverflow=off
  Check Within Limits : Subsystem
  Compare To Constant : simulink/Logic and Bit Operations/Compare To Constant  relop=<  const=2  OutDataTypeStr=boolean
  ElecToMechPwr : Product  Inputs=*/
  Mech to Elec Power Estimate : Subsystem
  MechPwrToTrq : Product  Inputs=*/
  Switch : Switch  Criteria=u2 > Threshold  SaturateOnIntegerOverflow=off  InputSameDT=off
  Switch1 : Switch  Criteria=u2 > Threshold  SaturateOnIntegerOverflow=off  InputSameDT=off
  Torque Limit : Subsystem
  div0protect - poly : autolibutils/div0protect - poly  thresh=2  ZeroCross1=on  aMode=aMode
  MotTrqCmdFinal : Outport  VectorParamsAs1DForOutWhenUnconnected=off
  wires:
  Compare To Constant/1 -> Switch1/2
  Abs/1 -> Compare To Constant/1
  Switch1/1 -> Torque Limit/1(MotTrq)
  Check Within Limits/1(InLimit) -> Switch/2
  Switch/1 -> Switch1/3
  Check Within Limits/2(y) -> ElecToMechPwr/1
  BattPwrChrgLmt/1 -> Check Within Limits/3(lo)
  Mech to Elec Power Estimate/1(MotPwrElecReq) -> Check Within Limits/2(u)
  BattPwrDischrgLmt/1 -> Check Within Limits/1(up)
  Torque Limit/1(MotTrqCmd) -> MotTrqCmdFinal/1
  MechPwrToTrq/1 -> Switch/3
  ElecToMechPwr/1 -> MechPwrToTrq/1
  Mech to Elec Power Estimate/2(Eff2k) -> ElecToMechPwr/2
  div0protect - poly/1 -> MechPwrToTrq/2
  MotTrqCmd/1 -> Mech to Elec Power Estimate/1(MotTrqCmd), Switch1/1, Switch/1
  MotSpd/1 -> Abs/1, Mech to Elec Power Estimate/2(MotSpd), div0protect - poly/1, Torque Limit/2(MotSpd)

== system CAVE_MachE_dSPACE_250912/Vehicle Under Test3/Vehicle/Rototest and ORNL Interface/From Rototest/RotoTestEthRX/Depacker ==
  SysStsBits : Inport
  Extract Bits1 : simulink/Logic and Bit Operations/Extract Bits  bitsToExtract=Range of bits  numBits=8  bitIdxRange=[7]  outScalingMode=Preserve fixed-point scaling
  Extract Bits10 : simulink/Logic and Bit Operations/Extract Bits  bitsToExtract=Range of bits  numBits=8  bitIdxRange=[9]  outScalingMode=Preserve fixed-point scaling
  Extract Bits11 : simulink/Logic and Bit Operations/Extract Bits  bitsToExtract=Range of bits  numBits=8  bitIdxRange=[10]  outScalingMode=Preserve fixed-point scaling
  Extract Bits12 : simulink/Logic and Bit Operations/Extract Bits  bitsToExtract=Range of bits  numBits=8  bitIdxRange=[11]  outScalingMode=Preserve fixed-point scaling
  Extract Bits13 : simulink/Logic and Bit Operations/Extract Bits  bitsToExtract=Range of bits  numBits=8  bitIdxRange=[12]  outScalingMode=Preserve fixed-point scaling
  Extract Bits14 : simulink/Logic and Bit Operations/Extract Bits  bitsToExtract=Range of bits  numBits=8  bitIdxRange=[13]  outScalingMode=Preserve fixed-point scaling
  Extract Bits15 : simulink/Logic and Bit Operations/Extract Bits  bitsToExtract=Range of bits  numBits=8  bitIdxRange=[14]  outScalingMode=Preserve fixed-point scaling
  Extract Bits16 : simulink/Logic and Bit Operations/Extract Bits  bitsToExtract=Range of bits  numBits=8  bitIdxRange=[15]  outScalingMode=Preserve fixed-point scaling
  Extract Bits2 : simulink/Logic and Bit Operations/Extract Bits  bitsToExtract=Range of bits  numBits=8  bitIdxRange=[6]  outScalingMode=Preserve fixed-point scaling
  Extract Bits3 : simulink/Logic and Bit Operations/Extract Bits  bitsToExtract=Range of bits  numBits=8  bitIdxRange=[5]  outScalingMode=Preserve fixed-point scaling
  Extract Bits4 : simulink/Logic and Bit Operations/Extract Bits  bitsToExtract=Range of bits  numBits=8  bitIdxRange=[4]  outScalingMode=Preserve fixed-point scaling
  Extract Bits5 : simulink/Logic and Bit Operations/Extract Bits  bitsToExtract=Range of bits  numBits=8  bitIdxRange=[3]  outScalingMode=Preserve fixed-point scaling
  Extract Bits6 : simulink/Logic and Bit Operations/Extract Bits  bitsToExtract=Range of bits  numBits=8  bitIdxRange=[2]  outScalingMode=Preserve fixed-point scaling
  Extract Bits7 : simulink/Logic and Bit Operations/Extract Bits  bitsToExtract=Range of bits  numBits=8  bitIdxRange=[1]  outScalingMode=Preserve fixed-point scaling
  Extract Bits8 : simulink/Logic and Bit Operations/Extract Bits  bitsToExtract=Range of bits  numBits=8  bitIdxRange=[0]  outScalingMode=Preserve fixed-point scaling
  Extract Bits9 : simulink/Logic and Bit Operations/Extract Bits  bitsToExtract=Range of bits  numBits=8  bitIdxRange=[8]  outScalingMode=Preserve fixed-point scaling
  Gain : Gain  Gain=1/128
  Gain1 : Gain  Gain=1/64
  Gain10 : Gain  Gain=1/1024
  Gain11 : Gain  Gain=1/2048
  Gain12 : Gain  Gain=1/4096
  Gain13 : Gain  Gain=1/8192
  Gain14 : Gain  Gain=1/16384
  Gain15 : Gain  Gain=1/32768
  Gain2 : Gain  Gain=1/32
  Gain3 : Gain  Gain=1/16
  Gain4 : Gain  Gain=1/8
  Gain5 : Gain  Gain=1/4
  Gain6 : Gain  Gain=1/2
  Gain7 : Gain  Gain=1/1
  Gain8 : Gain  Gain=1/256
  Gain9 : Gain  Gain=1/512
  Header : VSIGenLib/Header  not=''
  Terminator{,1..8} (9 alike) : Terminator
  FaultActive : Outport
  WarningsActive : Outport  Port=2
  SpTqRR : Outport  Port=3
  SpTqLR : Outport  Port=4
  SpTqRF : Outport  Port=5
  SpTqLF : Outport  Port=6
  SystemActive : Outport  Port=7
  wires:
  Gain5/1 -> Terminator3/1  "Reserved"
  Gain6/1 -> Terminator4/1  "Reserved"
  Gain3/1 -> Terminator1/1  "Reserved"
  Gain4/1 -> Terminator2/1  "Reserved"
  Gain2/1 -> Terminator/1  "Reserved"
  Gain1/1 -> WarningsActive/1  "WarningsActive"
  Gain/1 -> FaultActive/1  "FaultActive"
  Gain7/1 -> Terminator5/1  "Reserved"
  Gain8/1 -> SystemActive/1  "SystemActive"
  Gain9/1 -> SpTqLF/1  "SpTqLF"
  Gain10/1 -> SpTqRF/1  "SpTqRF"
  Gain11/1 -> SpTqLR/1  "SpTqLR"
  Gain12/1 -> SpTqRR/1  "SpTqRR"
  Gain14/1 -> Terminator7/1  "Reserved"
  Gain13/1 -> Terminator8/1  "Reserved"
  Gain15/1 -> Terminator6/1  "Reserved"
  SysStsBits/1 -> Extract Bits9/1, Extract Bits10/1, Extract Bits16/1, Extract Bits15/1, Extract Bits14/1, Extract Bits13/1, Extract Bits12/1, Extract Bits11/1, Extract Bits8/1, Extract Bits7/1, Extract Bits6/1, Extract Bits5/1, Extract Bits4/1, Extract Bits3/1, Extract Bits2/1, Extract Bits1/1
  Extract Bits16/1 -> Gain15/1
  Extract Bits14/1 -> Gain13/1
  Extract Bits15/1 -> Gain14/1
  Extract Bits13/1 -> Gain12/1
  Extract Bits12/1 -> Gain11/1
  Extract Bits11/1 -> Gain10/1
  Extract Bits9/1 -> Gain8/1
  Extract Bits10/1 -> Gain9/1
  Extract Bits2/1 -> Gain1/1
  Extract Bits5/1 -> Gain4/1
  Extract Bits1/1 -> Gain/1
  Extract Bits3/1 -> Gain2/1
  Extract Bits7/1 -> Gain6/1
  Extract Bits8/1 -> Gain7/1
  Extract Bits4/1 -> Gain3/1
  Extract Bits6/1 -> Gain5/1

== system CAVE_MachE_dSPACE_250912/Vehicle Under Test3/Vehicle/Rototest and ORNL Interface/Get Wheel Spd Cmd Based on Wheel Dynamics/Whl Dynamics & Format CM Powertrain Signal/Diff Trq ==
  In1 : Inport
  Constant : Constant  Value=4.1
  Gain10 : Gain  Gain=0.5
  Product : Product  RndMeth=Zero
  Out1 : Outport
  wires:
  Gain10/1 -> Out1/1
  Constant/1 -> Product/1
  In1/1 -> Product/2
  Product/1 -> Gain10/1  "DiffTrq"

== system CAVE_MachE_dSPACE_250912/Vehicle Under Test3/Vehicle/Rototest and ORNL Interface/Get Wheel Spd Cmd Based on Wheel Dynamics/Whl Dynamics & Format CM Powertrain Signal/Subsystem ==
  BrakeTorq : Inport
  <Car Trq_T2WFL> : Inport  Port=2
  AxlTorq : Inport  Port=3
  Fx : Inport  Port=4
  Add1 : Sum  Inputs=--+
  Add2 : Sum  Inputs=-+
  Constant : Constant  Value=0
  Constant9 : Constant  Value=0.3135
  MATLAB Function : MATLAB Function  TreatAsAtomicUnit=on
  Memory : Memory
  Output Damping : Gain  Gain=0  SaturateOnIntegerOverflow=on  OutDataTypeStr=Inherit: Same as input  ParamDataTypeStr=Inherit: Same as input
  Product3 : Product  Inputs=**
  Saturation : Saturate  UpperLimit=inf  LowerLimit=0  ZeroCross=off
  Sum : Sum  Inputs=--
  Sum3 : Sum  Inputs=-++
  Switch : Switch  Criteria=u2 > Threshold  SaturateOnIntegerOverflow=off  InputSameDT=off
  WheelInertia : Subsystem
  WheelInertia1 : Subsystem
  omega wheel : Integrator  ContinuousStateAttributes='omegaWheel'
  rotv FL : Outport
  wires:
  Sum3/1 -> WheelInertia/1(In1)
  BrakeTorq/1 -> Sum3/1
  MATLAB Function/1(switchFlag) -> Switch/2  "Flag1"
  Constant/1 -> Switch/1
  Memory/1 -> MATLAB Function/2(wheelSpd)
  Add2/1 -> Saturation/1
  [RhoZ1] -> Add2/1
  Constant9/1 -> Add2/2
  AxlTorq/1 -> Add1/1, MATLAB Function/1(axleTorq), Sum3/3
  <Car Trq_T2WFL>/1 -> Add1/2, Sum3/2
  Product3/1 -> Add1/3
  Saturation/1 -> Product3/2
  Add1/1 -> WheelInertia1/1(In1)
  Switch/1 -> omega wheel/1
  omega wheel/1 -> Memory/1, Output Damping/1, rotv FL/1
  Output Damping/1 -> Sum/2
  WheelInertia1/1(axleTorq) -> Sum/1  "rota"
  Sum/1 -> Switch/3
  [Fx1] -> Product3/1

== system CAVE_MachE_dSPACE_250912/Vehicle Under Test3/Vehicle/Rototest and ORNL Interface/Get Wheel Spd Cmd Based on Wheel Dynamics/Whl Dynamics & Format CM Powertrain Signal/Subsystem1 ==
  BrakeTorq : Inport
  <Car Trq_T2WFL> : Inport  Port=2
  AxlTorq : Inport  Port=3
  Discrete-Time Integrator : DiscreteIntegrator  IntegratorMethod=Integration: Backward Euler  InitialCondition=0/3.6/0.3235  SampleTime=0.001  ICPrevOutput=DiscIntNeverNeededParam  ICPrevScaledInput=DiscIntNeverNeededParam
  Sum3 : Sum  Inputs=-++
  WheelInertia : Subsystem
  rotv FL : Outport
  wires:
  Sum3/1 -> WheelInertia/1(In1)
  AxlTorq/1 -> Sum3/3
  <Car Trq_T2WFL>/1 -> Sum3/2
  BrakeTorq/1 -> Sum3/1
  Discrete-Time Integrator/1 -> rotv FL/1  "rotv FL"
  WheelInertia/1(Out1) -> Discrete-Time Integrator/1

== system CAVE_MachE_dSPACE_250912/Vehicle Under Test3/Vehicle/Rototest and ORNL Interface/Get Wheel Spd Cmd Based on Wheel Dynamics/Whl Dynamics & Format CM Powertrain Signal/Subsystem2 ==
  BrakeTorq : Inport
  <Car Trq_T2WFR> : Inport  Port=2
  AxlTorq : Inport  Port=3
  Fx : Inport  Port=4
  Add1 : Sum  Inputs=--+
  Add2 : Sum  Inputs=-+
  Constant : Constant  Value=0
  Constant9 : Constant  Value=0.3135
  MATLAB Function : MATLAB Function  TreatAsAtomicUnit=on
  Memory : Memory
  Output Damping : Gain  Gain=-1  SaturateOnIntegerOverflow=on  OutDataTypeStr=Inherit: Same as input  ParamDataTypeStr=Inherit: Same as input
  Product3 : Product  Inputs=**
  Saturation : Saturate  UpperLimit=inf  LowerLimit=0  ZeroCross=off
  Sum3 : Sum  Inputs=-++
  Switch : Switch  Criteria=u2 > Threshold  SaturateOnIntegerOverflow=off  InputSameDT=off
  WheelInertia : Subsystem
  WheelInertia1 : Subsystem
  omega wheel : Integrator  ContinuousStateAttributes='omegaWheel'
  rotv FR : Outport
  wires:
  MATLAB Function/1(switchFlag) -> Switch/2
  Constant/1 -> Switch/1
  BrakeTorq/1 -> Sum3/1
  Sum3/1 -> WheelInertia/1(In1)
  Memory/1 -> MATLAB Function/2(wheelSpd)
  WheelInertia1/1(Out1) -> Output Damping/1  "rota"
  Product3/1 -> Add1/3
  <Car Trq_T2WFR>/1 -> Add1/2, Sum3/2
  Constant9/1 -> Add2/2
  Add1/1 -> WheelInertia1/1(In1)
  [RhoZ2] -> Add2/1
  Saturation/1 -> Product3/2
  Add2/1 -> Saturation/1
  AxlTorq/1 -> Add1/1, MATLAB Function/1(axleTorq), Sum3/3
  omega wheel/1 -> Memory/1, rotv FR/1
  Switch/1 -> omega wheel/1
  Output Damping/1 -> Switch/3
  [Fx2] -> Product3/1

== system CAVE_MachE_dSPACE_250912/Vehicle Under Test3/Vehicle/Rototest and ORNL Interface/Get Wheel Spd Cmd Based on Wheel Dynamics/Whl Dynamics & Format CM Powertrain Signal/Subsystem3 ==
  BrakeTorq : Inport
  <Car Trq_T2WRL> : Inport  Port=2
  AxlTorq : Inport  Port=3
  Fx : Inport  Port=4
  FWSpd : Inport  Port=5
  Add1 : Sum  Inputs=--+
  Add2 : Sum  Inputs=-+
  Constant : Constant  Value=0
  Constant9 : Constant  Value=0.3135
  MATLAB Function : MATLAB Function  TreatAsAtomicUnit=on
  Memory : Memory
  Output Damping : Gain  Gain=0  SaturateOnIntegerOverflow=on  OutDataTypeStr=Inherit: Same as input  ParamDataTypeStr=Inherit: Same as input
  Product3 : Product  Inputs=**
  Saturation : Saturate  UpperLimit=inf  LowerLimit=0  ZeroCross=off
  Sum : Sum  Inputs=--
  Sum3 : Sum  Inputs=-++
  Switch : Switch  Criteria=u2 > Threshold  SaturateOnIntegerOverflow=off  InputSameDT=off
  WheelInertia : Subsystem
  WheelInertia1 : Subsystem
  omega wheel : Integrator  ContinuousStateAttributes='omegaWheel'
  rotv RL : Outport
  wires:
  MATLAB Function/1(switchFlag) -> Switch/2
  Constant/1 -> Switch/1
  BrakeTorq/1 -> Sum3/1
  Sum3/1 -> WheelInertia/1(In1)
  Product3/1 -> Add1/3
  <Car Trq_T2WRL>/1 -> Sum3/2, Add1/2
  Constant9/1 -> Add2/2
  Add1/1 -> WheelInertia1/1(In1)
  [RhoZ3] -> Add2/1
  Saturation/1 -> Product3/2
  Add2/1 -> Saturation/1
  AxlTorq/1 -> Add1/1, MATLAB Function/1(axleTorq), Sum3/3
  FWSpd/1 -> MATLAB Function/2(wheelSpd)
  Sum/1 -> Switch/3
  Switch/1 -> omega wheel/1
  [Fx3] -> Product3/1
  Output Damping/1 -> Sum/2
  omega wheel/1 -> Output Damping/1, rotv RL/1
  WheelInertia1/1(axleTorq) -> Sum/1  "rota"

== system CAVE_MachE_dSPACE_250912/Vehicle Under Test3/Vehicle/Rototest and ORNL Interface/Get Wheel Spd Cmd Based on Wheel Dynamics/Whl Dynamics & Format CM Powertrain Signal/Subsystem4 ==
  BrakeTorq : Inport
  <Car Trq_T2WRR> : Inport  Port=2
  AxlTorq : Inport  Port=3
  Fx : Inport  Port=4
  FWSpd : Inport  Port=5
  Add1 : Sum  Inputs=--+
  Add2 : Sum  Inputs=-+
  Constant : Constant  Value=0
  Constant9 : Constant  Value=0.3135
  Gain : Gain  Gain=-1
  MATLAB Function : MATLAB Function  TreatAsAtomicUnit=on
  Memory : Memory
  Product3 : Product  Inputs=**
  Saturation : Saturate  UpperLimit=inf  LowerLimit=0  ZeroCross=off
  Sum3 : Sum  Inputs=-++
  Switch : Switch  Criteria=u2 > Threshold  SaturateOnIntegerOverflow=off  InputSameDT=off
  WheelInertia : Subsystem
  WheelInertia1 : Subsystem
  omega wheel : Integrator  ContinuousStateAttributes='omegaWheel'
  rotv RR : Outport
  wires:
  MATLAB Function/1(switchFlag) -> Switch/2
  Constant/1 -> Switch/1
  BrakeTorq/1 -> Sum3/1
  Sum3/1 -> WheelInertia/1(In1)
  Product3/1 -> Add1/3
  <Car Trq_T2WRR>/1 -> Add1/2, Sum3/2
  Constant9/1 -> Add2/2
  Add1/1 -> WheelInertia1/1(In1)
  [RhoZ4] -> Add2/1
  Saturation/1 -> Product3/2
  Add2/1 -> Saturation/1
  AxlTorq/1 -> Add1/1, MATLAB Function/1(axleTorq), Sum3/3
  FWSpd/1 -> MATLAB Function/2(wheelSpd)
  Gain/1 -> Switch/3
  Switch/1 -> omega wheel/1
  omega wheel/1 -> rotv RR/1
  [Fx4] -> Product3/1
  WheelInertia1/1(axleTorq) -> Gain/1  "rota"

== system CAVE_MachE_dSPACE_250912/Vehicle Under Test3/Vehicle/Rototest and ORNL Interface/Get Wheel Spd Cmd Based on Wheel Dynamics/Whl Dynamics & Format CM Powertrain Signal/Subsystem5 ==
  In1 : Inport
  <Car Trq_T2WFR> : Inport  Port=2
  In3 : Inport  Port=3
  Discrete-Time Integrator1 : DiscreteIntegrator  IntegratorMethod=Integration: Backward Euler  InitialCondition=0/3.6/0.3235  SampleTime=0.001  ICPrevOutput=DiscIntNeverNeededParam  ICPrevScaledInput=DiscIntNeverNeededParam
  Sum2 : Sum  Inputs=-++
  WheelInertia1 : Subsystem
  rotv FR : Outport
  wires:
  <Car Trq_T2WFR>/1 -> Sum2/2
  Sum2/1 -> WheelInertia1/1(In1)
  In3/1 -> Sum2/3
  WheelInertia1/1(Out1) -> Discrete-Time Integrator1/1  "rota"
  In1/1 -> Sum2/1
  Discrete-Time Integrator1/1 -> rotv FR/1  "rotv FR"

== system CAVE_MachE_dSPACE_250912/Vehicle Under Test3/Vehicle/Rototest and ORNL Interface/Get Wheel Spd Cmd Based on Wheel Dynamics/Whl Dynamics & Format CM Powertrain Signal/Subsystem6 ==
  In1 : Inport
  <Car Trq_T2WRL> : Inport  Port=2
  In3 : Inport  Port=3
  Discrete-Time Integrator2 : DiscreteIntegrator  IntegratorMethod=Integration: Backward Euler  InitialCondition=0/3.6/0.3235  SampleTime=0.001  ICPrevOutput=DiscIntNeverNeededParam  ICPrevScaledInput=DiscIntNeverNeededParam
  Sum : Sum  Inputs=-++
  WheelInertia2 : Subsystem
  rotv RL : Outport
  wires:
  In3/1 -> Sum/3
  WheelInertia2/1(Out1) -> Discrete-Time Integrator2/1  "rota"
  <Car Trq_T2WRL>/1 -> Sum/2
  Sum/1 -> WheelInertia2/1(In1)
  Discrete-Time Integrator2/1 -> rotv RL/1  "rotv RL"
  In1/1 -> Sum/1

== system CAVE_MachE_dSPACE_250912/Vehicle Under Test3/Vehicle/Rototest and ORNL Interface/Get Wheel Spd Cmd Based on Wheel Dynamics/Whl Dynamics & Format CM Powertrain Signal/Subsystem7 ==
  In1 : Inport
  <Car Trq_T2WRR> : Inport  Port=2
  In3 : Inport  Port=3
  Discrete-Time Integrator3 : DiscreteIntegrator  IntegratorMethod=Integration: Backward Euler  InitialCondition=0/3.6/0.3235  SampleTime=0.001  ICPrevOutput=DiscIntNeverNeededParam  ICPrevScaledInput=DiscIntNeverNeededParam
  Sum1 : Sum  Inputs=-++
  WheelInertia3 : Subsystem
  rotv RR : Outport
  wires:
  Sum1/1 -> WheelInertia3/1(In1)
  WheelInertia3/1(Out1) -> Discrete-Time Integrator3/1  "rota"
  In3/1 -> Sum1/3
  <Car Trq_T2WRR>/1 -> Sum1/2
  In1/1 -> Sum1/1
  Discrete-Time Integrator3/1 -> rotv RR/1  "rotv RR"
